simulink model "powertrain_wip_myBatt"  (R2019a)
settings: Solver=VariableStepAuto  StartTime=0.0  StopTime=100  FixedStep=.001  RelTol=1e-3
values from neighbouring files (symbols this model uses):
  Motor =     [current.mat]    (also in rpm.mat; thrust.mat; tout.mat)
undefined symbols (not defined in the file or in its folder): quadModel
libraries: simulink x8
settings Model: Creator=tdarrah  LastModifiedBy=tdarrah
settings DebuggingCC: ArithmeticOperatorsInVariantConditions=warning

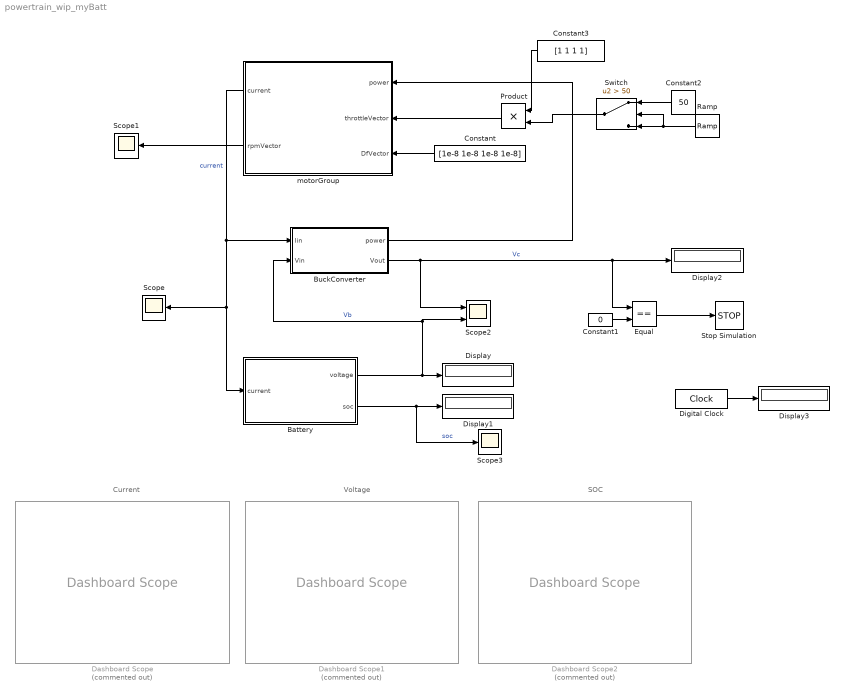
== system powertrain_wip_myBatt ==
  note: Current
  note: Voltage
  note: SOC
  Battery : Subsystem
  BuckConverter : Subsystem
  Constant : Constant  Value=[1e-8 1e-8 1e-8 1e-8]
  Constant1 : Constant  Value=0
  Constant2 : Constant  Value=50
  Constant3 : Constant  Value=[1 1 1 1]
  Dashboard Scope : DashboardScope  Commented=on  Ymin=-5  Ymax=10
  Dashboard Scope1 : DashboardScope  Commented=on  Ymin=8  Ymax=13
  Dashboard Scope2 : DashboardScope  Commented=on
  Digital Clock : DigitalClock
      mask Display: disp('Sim Time');
  Display{,1..3} (4 alike) : Display
  Equal : RelationalOperator  Operator===  OutDataTypeStr=boolean  RndMeth=Simplest
  Product : Product
  Ramp : simulink/Sources/Ramp  slope=1  start=0  InitialOutput=0
  Scope : Scope
  Scope1 : Scope
  Scope2 : Scope  NumInputPorts=2
  Scope3 : Scope
  Stop Simulation : Stop
  Switch : Switch  Criteria=u2 > Threshold  Threshold=50
  motorGroup : Subsystem
  wires:
  Battery/1(voltage) -> BuckConverter/2(Vin), Scope2/2, Display/1  "Vb"
  Battery/2(soc) -> Scope3/1, Display1/1  "soc"
  motorGroup/1(current) -> BuckConverter/1(Iin), Battery/1(current), Scope/1  "current"
  BuckConverter/1(power) -> motorGroup/1(power)
  BuckConverter/2(Vout) -> Scope2/1, Equal/1, Display2/1  "Vc"
  Product/1 -> motorGroup/2(throttleVector)
  Constant/1 -> motorGroup/3(DfVector)
  motorGroup/2(rpmVector) -> Scope1/1
  Constant1/1 -> Equal/2
  Equal/1 -> Stop Simulation/1
  Digital Clock/1 -> Display3/1
  Ramp/1 -> Switch/2, Switch/3
  Constant2/1 -> Switch/1
  Constant3/1 -> Product/1
  Switch/1 -> Product/2

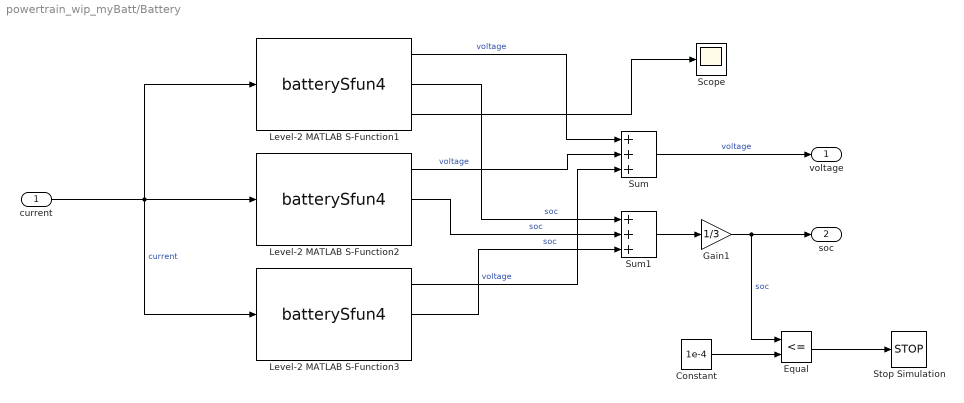
== system powertrain_wip_myBatt/Battery ==
  current : Inport
  Constant : Constant  Value=1e-4
  Equal : RelationalOperator  Operator=<=  OutDataTypeStr=boolean  RndMeth=Simplest
  Gain1 : Gain  Gain=1/3
  Level-2 MATLAB S-Function1 : M-S-Function  FunctionName=batterySfun4  Parameters=battery, soc_ocv, .001
      mask Display:
      | port_label('input', 1, 'current');
      | port_label('output', 1, 'voltage');
      | port_label('output', 2, 'soc');
  Level-2 MATLAB S-Function2 : M-S-Function  FunctionName=batterySfun4  Parameters=battery, soc_ocv, .001
      mask Display:
      | port_label('input', 1, 'current');
      | port_label('output', 1, 'voltage');
      | port_label('output', 2, 'soc');
  Level-2 MATLAB S-Function3 : M-S-Function  FunctionName=batterySfun4  Parameters=battery, soc_ocv, .001
      mask Display:
      | port_label('input', 1, 'current');
      | port_label('output', 1, 'voltage');
      | port_label('output', 2, 'soc');
  Scope : Scope
  Stop Simulation : Stop
  Sum : Sum  Inputs=+++
  Sum1 : Sum  Inputs=+++
  voltage : Outport
  soc : Outport  Port=2
  wires:
  Level-2 MATLAB S-Function2/1 -> Sum/2  "voltage"
  Level-2 MATLAB S-Function1/1 -> Sum/1  "voltage"
  Level-2 MATLAB S-Function2/2 -> Sum1/2  "soc"
  Sum1/1 -> Gain1/1
  Gain1/1 -> Equal/1, soc/1  "soc"
  Level-2 MATLAB S-Function1/2 -> Sum1/1  "soc"
  Level-2 MATLAB S-Function3/2 -> Sum1/3  "soc"
  current/1 -> Level-2 MATLAB S-Function3/1, Level-2 MATLAB S-Function1/1, Level-2 MATLAB S-Function2/1  "current"
  Level-2 MATLAB S-Function3/1 -> Sum/3  "voltage"
  Sum/1 -> voltage/1  "voltage"
  Level-2 MATLAB S-Function1/3 -> Scope/1
  Constant/1 -> Equal/2
  Equal/1 -> Stop Simulation/1

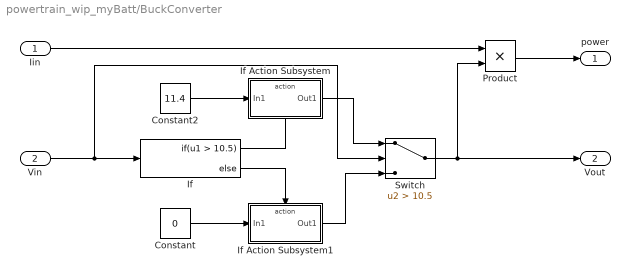
== system powertrain_wip_myBatt/BuckConverter ==
  Iin : Inport
  Vin : Inport  Port=2
  Constant : Constant  Value=0
  Constant2 : Constant  Value=11.4
  If : If  IfExpression=u1 > 10.5
  If Action Subsystem : Subsystem  TreatAsAtomicUnit=on
  If Action Subsystem1 : Subsystem  TreatAsAtomicUnit=on
  Product : Product
  Switch : Switch  Criteria=u2 > Threshold  Threshold=10.5
  power : Outport
  Vout : Outport  Port=2
  wires:
  Product/1 -> power/1
  Iin/1 -> Product/1
  If/1 -> If Action Subsystem/Action
  If/2 -> If Action Subsystem1/Action
  Constant/1 -> If Action Subsystem1/1(In1)
  If Action Subsystem/1(Out1) -> Switch/1
  If Action Subsystem1/1(Out1) -> Switch/3
  Constant2/1 -> If Action Subsystem/1(In1)
  Vin/1 -> Switch/2, If/1
  Switch/1 -> Product/2, Vout/1

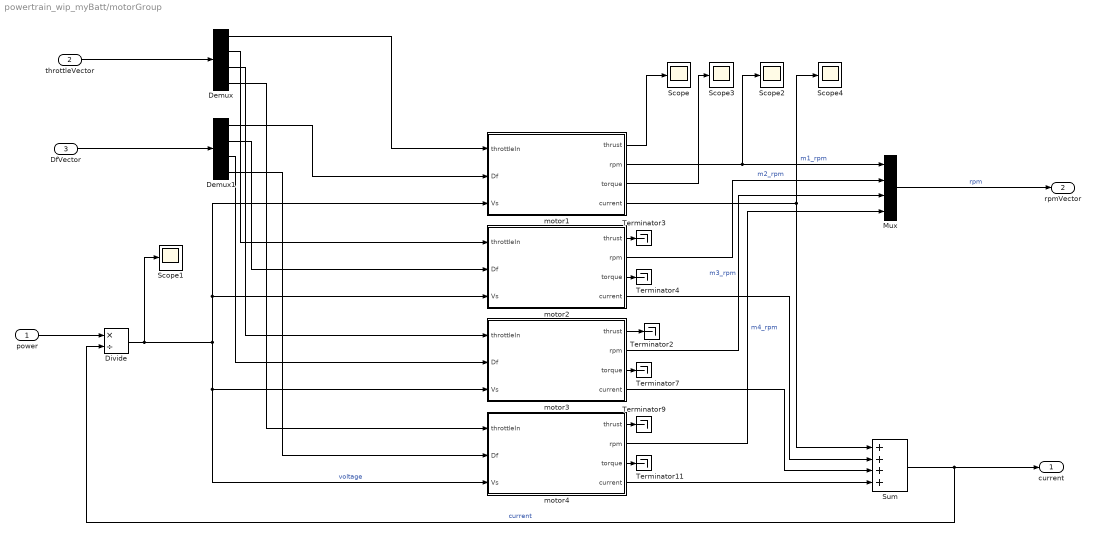
== system powertrain_wip_myBatt/motorGroup ==
  power : Inport
  throttleVector : Inport  Port=2  PortDimensions=4
  DfVector : Inport  Port=3  PortDimensions=4
  Demux : Demux
  Demux1 : Demux
  Divide : Product  Inputs=*/
  Mux : Mux
  Scope{,1..4} (5 alike) : Scope
  Sum : Sum  Inputs=++++
  Terminator{2..4,7,9,11} (6 alike) : Terminator
  motor1 : Subsystem
  motor2 : Subsystem
  motor3 : Subsystem
  motor4 : Subsystem
  current : Outport
  rpmVector : Outport  Port=2
  wires:
  Demux1/2 -> motor2/2(Df)
  Demux1/4 -> motor4/2(Df)
  Divide/1 -> Scope1/1, motor1/3(Vs), motor2/3(Vs), motor4/3(Vs), motor3/3(Vs)  "voltage"
  Demux1/1 -> motor1/2(Df)
  Sum/1 -> current/1, Divide/2  "current"
  Demux1/3 -> motor3/2(Df)
  motor1/4(current) -> Scope4/1, Sum/1
  power/1 -> Divide/1
  Demux/4 -> motor4/1(throttleIn)
  Demux/3 -> motor3/1(throttleIn)
  Demux/2 -> motor2/1(throttleIn)
  Demux/1 -> motor1/1(throttleIn)
  throttleVector/1 -> Demux/1
  DfVector/1 -> Demux1/1
  motor4/4(current) -> Sum/4
  motor3/4(current) -> Sum/3
  motor2/4(current) -> Sum/2
  motor4/2(rpm) -> Mux/4  "m4_rpm"
  motor3/2(rpm) -> Mux/3  "m3_rpm"
  motor2/2(rpm) -> Mux/2  "m2_rpm"
  motor1/2(rpm) -> Scope2/1, Mux/1  "m1_rpm"
  Mux/1 -> rpmVector/1  "rpm"
  motor1/1(thrust) -> Scope/1
  motor4/3(torque) -> Terminator11/1
  motor1/3(torque) -> Scope3/1
  motor2/3(torque) -> Terminator4/1
  motor3/3(torque) -> Terminator7/1
  motor4/1(thrust) -> Terminator9/1
  motor3/1(thrust) -> Terminator2/1
  motor2/1(thrust) -> Terminator3/1

== system powertrain_wip_myBatt/BuckConverter/If Action Subsystem ==
  In1 : Inport
  Action Port : ActionPort  ActionPortLabel=if(u1 > 10.5)
  Out1 : Outport
  wires:
  In1/1 -> Out1/1

== system powertrain_wip_myBatt/BuckConverter/If Action Subsystem1 ==
  In1 : Inport
  Action Port : ActionPort  ActionPortLabel=else
  Out1 : Outport
  wires:
  In1/1 -> Out1/1

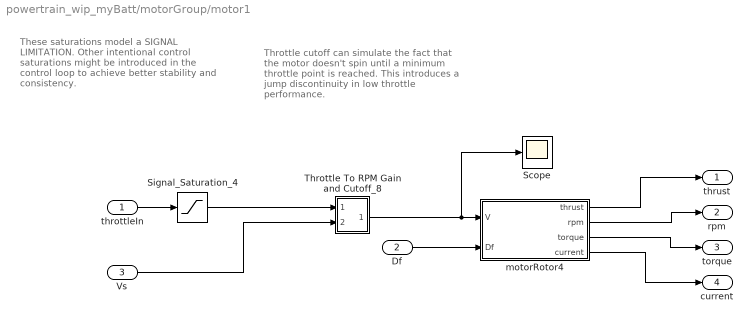
== system powertrain_wip_myBatt/motorGroup/motor1 ==
  note: Throttle cutoff can simulate the fact that the motor doesn't
      | spin until a minimum throttle point is reached. This introduces
      | a jump discontinuity in low throttle performance.
  note: These saturations model a SIGNAL LIMITATION.
      | Other intentional control saturations might be introduced in the
      | control loop to achieve better stability and consistency.
  throttleIn : Inport
  Df : Inport  Port=2
  Vs : Inport  Port=3
  Scope : Scope
  Signal_Saturation_4 : Saturate  UpperLimit=100  LowerLimit=0
  Throttle To RPM Gain and Cutoff_8 : Subsystem
  motorRotor4 : Subsystem
  thrust : Outport
  rpm : Outport  Port=2
  torque : Outport  Port=3
  current : Outport  Port=4
  wires:
  Throttle To RPM Gain and Cutoff_8/1(Out5) -> motorRotor4/1(V), Scope/1
  motorRotor4/4(current) -> current/1
  motorRotor4/2(rpm) -> rpm/1
  throttleIn/1 -> Signal_Saturation_4/1
  motorRotor4/3(torque) -> torque/1
  motorRotor4/1(thrust) -> thrust/1
  Signal_Saturation_4/1 -> Throttle To RPM Gain and Cutoff_8/1(In5)
  Df/1 -> motorRotor4/2(Df)
  Vs/1 -> Throttle To RPM Gain and Cutoff_8/2(Vs)

== system powertrain_wip_myBatt/motorGroup/motor2 ==
  note: Throttle cutoff can simulate the fact that the motor doesn't
      | spin until a minimum throttle point is reached. This introduces
      | a jump discontinuity in low throttle performance.
  note: These saturations model a SIGNAL LIMITATION.
      | Other intentional control saturations might be introduced in the
      | control loop to achieve better stability and consistency.
  throttleIn : Inport
  Df : Inport  Port=2
  Vs : Inport  Port=3
  Scope : Scope
  Signal_Saturation_4 : Saturate  UpperLimit=100  LowerLimit=0
  Throttle To RPM Gain and Cutoff_8 : Subsystem
  motorRotor4 : Subsystem
  thrust : Outport
  rpm : Outport  Port=2
  torque : Outport  Port=3
  current : Outport  Port=4
  wires:
  Throttle To RPM Gain and Cutoff_8/1(Out5) -> motorRotor4/1(V), Scope/1
  motorRotor4/4(current) -> current/1
  motorRotor4/2(rpm) -> rpm/1
  throttleIn/1 -> Signal_Saturation_4/1
  motorRotor4/3(torque) -> torque/1
  motorRotor4/1(thrust) -> thrust/1
  Signal_Saturation_4/1 -> Throttle To RPM Gain and Cutoff_8/1(In5)
  Df/1 -> motorRotor4/2(Df)
  Vs/1 -> Throttle To RPM Gain and Cutoff_8/2(Vs)

== system powertrain_wip_myBatt/motorGroup/motor3 ==
  note: Throttle cutoff can simulate the fact that the motor doesn't
      | spin until a minimum throttle point is reached. This introduces
      | a jump discontinuity in low throttle performance.
  note: These saturations model a SIGNAL LIMITATION.
      | Other intentional control saturations might be introduced in the
      | control loop to achieve better stability and consistency.
  throttleIn : Inport
  Df : Inport  Port=2
  Vs : Inport  Port=3
  Scope : Scope
  Signal_Saturation_4 : Saturate  UpperLimit=100  LowerLimit=0
  Throttle To RPM Gain and Cutoff_8 : Subsystem
  motorRotor4 : Subsystem
  thrust : Outport
  rpm : Outport  Port=2
  torque : Outport  Port=3
  current : Outport  Port=4
  wires:
  Throttle To RPM Gain and Cutoff_8/1(Out5) -> motorRotor4/1(V), Scope/1
  motorRotor4/4(current) -> current/1
  motorRotor4/2(rpm) -> rpm/1
  throttleIn/1 -> Signal_Saturation_4/1
  motorRotor4/3(torque) -> torque/1
  motorRotor4/1(thrust) -> thrust/1
  Signal_Saturation_4/1 -> Throttle To RPM Gain and Cutoff_8/1(In5)
  Df/1 -> motorRotor4/2(Df)
  Vs/1 -> Throttle To RPM Gain and Cutoff_8/2(Vs)

== system powertrain_wip_myBatt/motorGroup/motor4 ==
  note: Throttle cutoff can simulate the fact that the motor doesn't
      | spin until a minimum throttle point is reached. This introduces
      | a jump discontinuity in low throttle performance.
  note: These saturations model a SIGNAL LIMITATION.
      | Other intentional control saturations might be introduced in the
      | control loop to achieve better stability and consistency.
  throttleIn : Inport
  Df : Inport  Port=2
  Vs : Inport  Port=3
  Scope : Scope
  Signal_Saturation_4 : Saturate  UpperLimit=100  LowerLimit=0
  Throttle To RPM Gain and Cutoff_8 : Subsystem
  motorRotor4 : Subsystem
  thrust : Outport
  rpm : Outport  Port=2
  torque : Outport  Port=3
  current : Outport  Port=4
  wires:
  Throttle To RPM Gain and Cutoff_8/1(Out5) -> motorRotor4/1(V), Scope/1
  motorRotor4/4(current) -> current/1
  motorRotor4/2(rpm) -> rpm/1
  throttleIn/1 -> Signal_Saturation_4/1
  motorRotor4/3(torque) -> torque/1
  motorRotor4/1(thrust) -> thrust/1
  Signal_Saturation_4/1 -> Throttle To RPM Gain and Cutoff_8/1(In5)
  Df/1 -> motorRotor4/2(Df)
  Vs/1 -> Throttle To RPM Gain and Cutoff_8/2(Vs)

== system powertrain_wip_myBatt/motorGroup/motor1/Throttle To RPM Gain and Cutoff_8 ==
  note: Output equals linearly scaled RPM
      | for given throttle input if throttle input >=Throttle Cuttoff (minThr)
      | else output is zero.
  In5 : Inport
  Vs : Inport  Port=2
  Gain : Gain  Gain=.01
  Minimum Throttle Cutoff : simulink/Logic and Bit Operations/Compare To Constant  relop=>=  const=5  OutDataTypeStr=uint8
  Product : Product
  Product2 : Product
  Out5 : Outport
  wires:
  Minimum Throttle Cutoff/1 -> Product/2
  Product/1 -> Out5/1
  In5/1 -> Gain/1, Minimum Throttle Cutoff/1
  Gain/1 -> Product2/2
  Product2/1 -> Product/1
  Vs/1 -> Product2/1

== system powertrain_wip_myBatt/motorGroup/motor1/motorRotor4 ==
  V : Inport
  Df : Inport  Port=2
  Electrical part : Subsystem
  Mechanical part : Subsystem
  thrust : Outport
  rpm : Outport  Port=2
  torque : Outport  Port=3
  current : Outport  Port=4
  wires:
  V/1 -> Electrical part/1(Vin)
  Mechanical part/2(Thrust) -> thrust/1
  Electrical part/1(Electrical Torque) -> Mechanical part/2(Electrical Torque)
  Mechanical part/4(Torque) -> torque/1
  Mechanical part/1(w angular speed) -> Electrical part/2(w angular speed)
  Df/1 -> Mechanical part/1(dynamicFriction)
  Electrical part/2(current) -> current/1
  Mechanical part/3(rpm) -> rpm/1

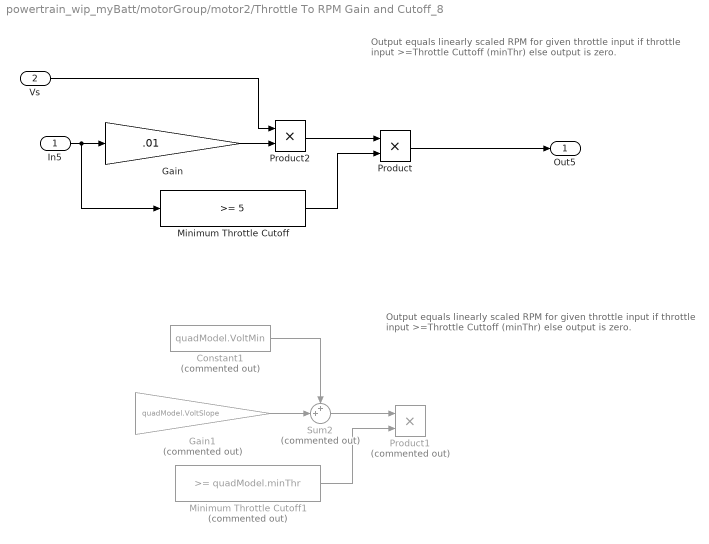
== system powertrain_wip_myBatt/motorGroup/motor2/Throttle To RPM Gain and Cutoff_8 ==
  note: Output equals linearly scaled RPM
      | for given throttle input if throttle input >=Throttle Cuttoff (minThr)
      | else output is zero.
  note: Output equals linearly scaled RPM
      | for given throttle input if throttle input >=Throttle Cuttoff (minThr)
      | else output is zero.
  In5 : Inport
  Vs : Inport  Port=2
  Constant1 : Constant  Commented=on  Value=quadModel.VoltMin
  Gain : Gain  Gain=.01
  Gain1 : Gain  Commented=on  Gain=quadModel.VoltSlope
  Minimum Throttle Cutoff : simulink/Logic and Bit Operations/Compare To Constant  relop=>=  const=5  OutDataTypeStr=uint8
  Minimum Throttle Cutoff1 : simulink/Logic and Bit Operations/Compare To Constant  Commented=on  relop=>=  const=quadModel.minThr  OutDataTypeStr=uint8
  Product : Product
  Product1 : Product  Commented=on
  Product2 : Product
  Sum2 : Sum  Commented=on  Inputs=++|
  Out5 : Outport
  wires:
  Minimum Throttle Cutoff/1 -> Product/2
  Product/1 -> Out5/1
  In5/1 -> Gain/1, Minimum Throttle Cutoff/1
  Gain/1 -> Product2/2
  Product2/1 -> Product/1
  Gain1/1 -> Sum2/2
  Constant1/1 -> Sum2/1
  Sum2/1 -> Product1/1
  Minimum Throttle Cutoff1/1 -> Product1/2
  Vs/1 -> Product2/1

== system powertrain_wip_myBatt/motorGroup/motor2/motorRotor4 ==
  V : Inport
  Df : Inport  Port=2
  Convert rad/s to rmp : Gain  Gain=60/(2*pi)
  Electrical part : Subsystem
  Mechanical part : Subsystem
  thrust : Outport
  rpm : Outport  Port=2
  torque : Outport  Port=3
  current : Outport  Port=4
  wires:
  Convert rad/s to rmp/1 -> rpm/1
  V/1 -> Electrical part/1(ESC voltage)
  Mechanical part/2(Thrust) -> thrust/1
  Electrical part/1(Electrical Torque) -> Mechanical part/2(Electrical Torque)
  Mechanical part/3(Torque) -> torque/1
  Mechanical part/1(w angular speed) -> Electrical part/2(w angular speed), Convert rad/s to rmp/1
  Df/1 -> Mechanical part/1(dynamicFriction)
  Electrical part/2(current) -> current/1

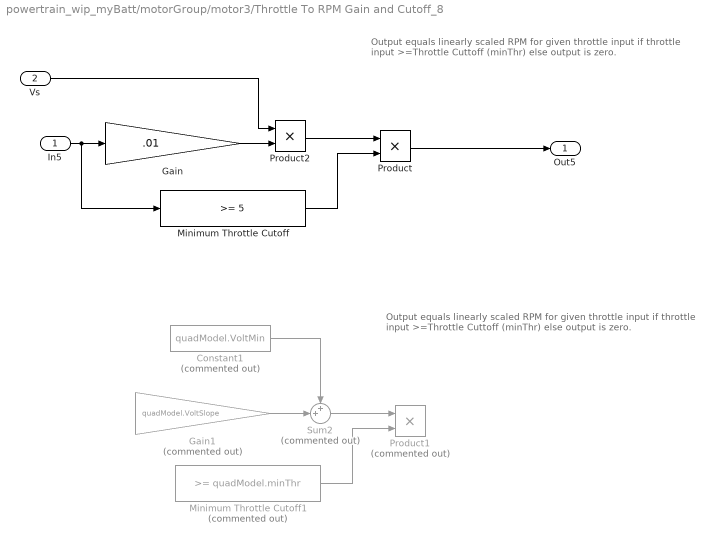
== system powertrain_wip_myBatt/motorGroup/motor3/Throttle To RPM Gain and Cutoff_8 ==
  note: Output equals linearly scaled RPM
      | for given throttle input if throttle input >=Throttle Cuttoff (minThr)
      | else output is zero.
  note: Output equals linearly scaled RPM
      | for given throttle input if throttle input >=Throttle Cuttoff (minThr)
      | else output is zero.
  In5 : Inport
  Vs : Inport  Port=2
  Constant1 : Constant  Commented=on  Value=quadModel.VoltMin
  Gain : Gain  Gain=.01
  Gain1 : Gain  Commented=on  Gain=quadModel.VoltSlope
  Minimum Throttle Cutoff : simulink/Logic and Bit Operations/Compare To Constant  relop=>=  const=5  OutDataTypeStr=uint8
  Minimum Throttle Cutoff1 : simulink/Logic and Bit Operations/Compare To Constant  Commented=on  relop=>=  const=quadModel.minThr  OutDataTypeStr=uint8
  Product : Product
  Product1 : Product  Commented=on
  Product2 : Product
  Sum2 : Sum  Commented=on  Inputs=++|
  Out5 : Outport
  wires:
  Minimum Throttle Cutoff/1 -> Product/2
  Product/1 -> Out5/1
  In5/1 -> Gain/1, Minimum Throttle Cutoff/1
  Gain/1 -> Product2/2
  Product2/1 -> Product/1
  Gain1/1 -> Sum2/2
  Constant1/1 -> Sum2/1
  Sum2/1 -> Product1/1
  Minimum Throttle Cutoff1/1 -> Product1/2
  Vs/1 -> Product2/1

== system powertrain_wip_myBatt/motorGroup/motor3/motorRotor4 ==
  V : Inport
  Df : Inport  Port=2
  Convert rad/s to rmp : Gain  Gain=60/(2*pi)
  Electrical part : Subsystem
  Mechanical part : Subsystem
  thrust : Outport
  rpm : Outport  Port=2
  torque : Outport  Port=3
  current : Outport  Port=4
  wires:
  Convert rad/s to rmp/1 -> rpm/1
  V/1 -> Electrical part/1(ESC voltage)
  Mechanical part/2(Thrust) -> thrust/1
  Electrical part/1(Electrical Torque) -> Mechanical part/2(Electrical Torque)
  Mechanical part/3(Torque) -> torque/1
  Mechanical part/1(w angular speed) -> Electrical part/2(w angular speed), Convert rad/s to rmp/1
  Df/1 -> Mechanical part/1(dynamicFriction)
  Electrical part/2(current) -> current/1

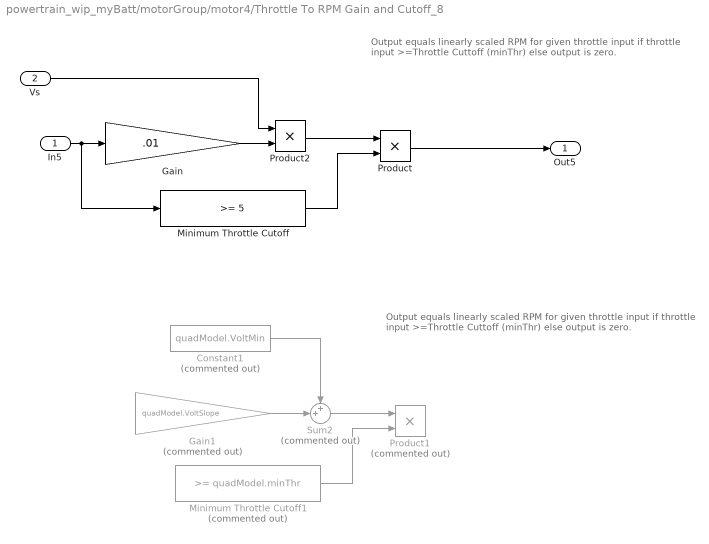
== system powertrain_wip_myBatt/motorGroup/motor4/Throttle To RPM Gain and Cutoff_8 ==
  note: Output equals linearly scaled RPM
      | for given throttle input if throttle input >=Throttle Cuttoff (minThr)
      | else output is zero.
  note: Output equals linearly scaled RPM
      | for given throttle input if throttle input >=Throttle Cuttoff (minThr)
      | else output is zero.
  In5 : Inport
  Vs : Inport  Port=2
  Constant1 : Constant  Commented=on  Value=quadModel.VoltMin
  Gain : Gain  Gain=.01
  Gain1 : Gain  Commented=on  Gain=quadModel.VoltSlope
  Minimum Throttle Cutoff : simulink/Logic and Bit Operations/Compare To Constant  relop=>=  const=5  OutDataTypeStr=uint8
  Minimum Throttle Cutoff1 : simulink/Logic and Bit Operations/Compare To Constant  Commented=on  relop=>=  const=quadModel.minThr  OutDataTypeStr=uint8
  Product : Product
  Product1 : Product  Commented=on
  Product2 : Product
  Sum2 : Sum  Commented=on  Inputs=++|
  Out5 : Outport
  wires:
  Minimum Throttle Cutoff/1 -> Product/2
  Product/1 -> Out5/1
  In5/1 -> Gain/1, Minimum Throttle Cutoff/1
  Gain/1 -> Product2/2
  Product2/1 -> Product/1
  Gain1/1 -> Sum2/2
  Constant1/1 -> Sum2/1
  Sum2/1 -> Product1/1
  Minimum Throttle Cutoff1/1 -> Product1/2
  Vs/1 -> Product2/1

== system powertrain_wip_myBatt/motorGroup/motor4/motorRotor4 ==
  V : Inport
  Df : Inport  Port=2
  Convert rad/s to rmp : Gain  Gain=60/(2*pi)
  Electrical part : Subsystem
  Mechanical part : Subsystem
  thrust : Outport
  rpm : Outport  Port=2
  torque : Outport  Port=3
  current : Outport  Port=4
  wires:
  Convert rad/s to rmp/1 -> rpm/1
  V/1 -> Electrical part/1(ESC voltage)
  Mechanical part/2(Thrust) -> thrust/1
  Electrical part/1(Electrical Torque) -> Mechanical part/2(Electrical Torque)
  Mechanical part/3(Torque) -> torque/1
  Mechanical part/1(w angular speed) -> Electrical part/2(w angular speed), Convert rad/s to rmp/1
  Df/1 -> Mechanical part/1(dynamicFriction)
  Electrical part/2(current) -> current/1

== system powertrain_wip_myBatt/motorGroup/motor1/motorRotor4/Electrical part ==
  Vin : Inport
  w angular speed : Inport  Port=2
  1/R : Gain  Gain=1/Motor.Req
  Ke (Torque constant)1 : Gain  Gain=Motor.Ke_eq
  Kt (Torque constant) Kt=Ke for an ideal square wave motor : Gain  Gain=Motor.Ke_eq
  Sum : Sum  Inputs=|+-
  Electrical Torque : Outport
  current : Outport  Port=2
  wires:
  1/R/1 -> current/1, Kt (Torque constant) Kt=Ke for an ideal square wave motor/1  "current i"
  Sum/1 -> 1/R/1
  Kt (Torque constant) Kt=Ke for an ideal square wave motor/1 -> Electrical Torque/1
  Ke (Torque constant)1/1 -> Sum/2
  Vin/1 -> Sum/1
  w angular speed/1 -> Ke (Torque constant)1/1

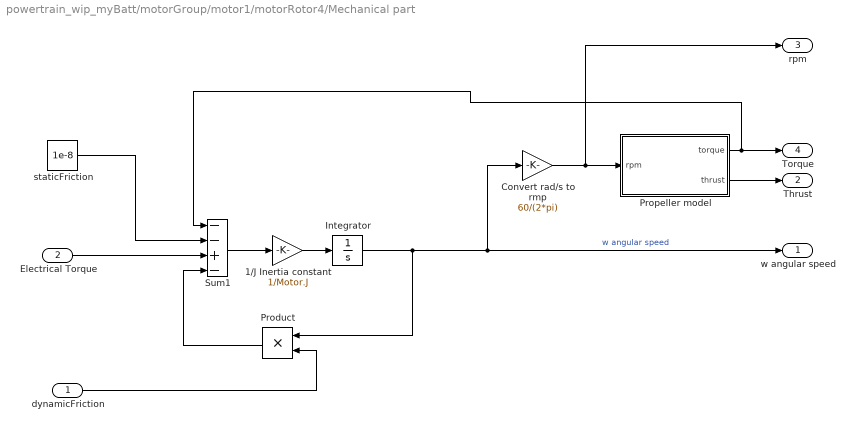
== system powertrain_wip_myBatt/motorGroup/motor1/motorRotor4/Mechanical part ==
  dynamicFriction : Inport
  Electrical Torque : Inport  Port=2
  1/J Inertia constant : Gain  Gain=1/Motor.J
  Convert rad/s to rmp : Gain  Gain=60/(2*pi)
  Integrator : Integrator  InitialCondition=419
  Product : Product
  "Propeller model " : MATLAB Function  TreatAsAtomicUnit=on
  Sum1 : Sum  Inputs=--+-
  staticFriction : Constant  Value=1e-8
  w angular speed : Outport
  Thrust : Outport  Port=2
  rpm : Outport  Port=3
  Torque : Outport  Port=4
  wires:
  "Propeller model "/1(torque) -> Sum1/1, Torque/1
  1/J Inertia constant/1 -> Integrator/1
  dynamicFriction/1 -> Product/2
  Product/1 -> Sum1/4
  Integrator/1 -> Product/1, w angular speed/1, Convert rad/s to rmp/1  "w angular speed"
  Sum1/1 -> 1/J Inertia constant/1
  Electrical Torque/1 -> Sum1/3
  Convert rad/s to rmp/1 -> rpm/1, "Propeller model "/1(rpm)
  "Propeller model "/2(thrust) -> Thrust/1
  staticFriction/1 -> Sum1/2

== system powertrain_wip_myBatt/motorGroup/motor2/motorRotor4/Electrical part ==
  ESC voltage : Inport
  w angular speed : Inport  Port=2
  1/R : Gain  Gain=1/Motor.Req
  Ke (Torque constant)1 : Gain  Gain=Motor.Ke_eq
  Kt (Torque constant) Kt=Ke for an ideal square wave motor : Gain  Gain=Motor.Ke_eq
  Sum : Sum  Inputs=|+-
  Electrical Torque : Outport
  current : Outport  Port=2
  wires:
  1/R/1 -> current/1, Kt (Torque constant) Kt=Ke for an ideal square wave motor/1  "current i"
  Sum/1 -> 1/R/1
  Kt (Torque constant) Kt=Ke for an ideal square wave motor/1 -> Electrical Torque/1
  Ke (Torque constant)1/1 -> Sum/2
  ESC voltage/1 -> Sum/1
  w angular speed/1 -> Ke (Torque constant)1/1

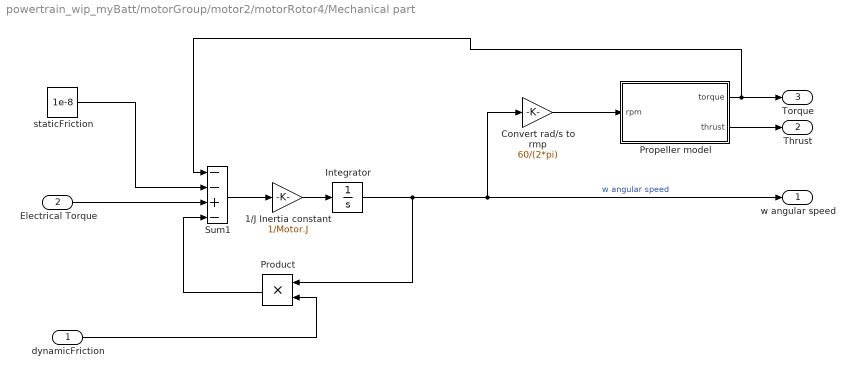
== system powertrain_wip_myBatt/motorGroup/motor2/motorRotor4/Mechanical part ==
  dynamicFriction : Inport
  Electrical Torque : Inport  Port=2
  1/J Inertia constant : Gain  Gain=1/Motor.J
  Convert rad/s to rmp : Gain  Gain=60/(2*pi)
  Integrator : Integrator  InitialCondition=419
  Product : Product
  "Propeller model " : MATLAB Function  TreatAsAtomicUnit=on
  Sum1 : Sum  Inputs=--+-
  staticFriction : Constant  Value=1e-8
  w angular speed : Outport
  Thrust : Outport  Port=2
  Torque : Outport  Port=3
  wires:
  "Propeller model "/1(torque) -> Sum1/1, Torque/1
  1/J Inertia constant/1 -> Integrator/1
  dynamicFriction/1 -> Product/2
  Product/1 -> Sum1/4
  Integrator/1 -> Product/1, w angular speed/1, Convert rad/s to rmp/1  "w angular speed"
  Sum1/1 -> 1/J Inertia constant/1
  Electrical Torque/1 -> Sum1/3
  Convert rad/s to rmp/1 -> "Propeller model "/1(rpm)
  "Propeller model "/2(thrust) -> Thrust/1
  staticFriction/1 -> Sum1/2

== system powertrain_wip_myBatt/motorGroup/motor3/motorRotor4/Electrical part ==
  ESC voltage : Inport
  w angular speed : Inport  Port=2
  1/R : Gain  Gain=1/Motor.Req
  Ke (Torque constant)1 : Gain  Gain=Motor.Ke_eq
  Kt (Torque constant) Kt=Ke for an ideal square wave motor : Gain  Gain=Motor.Ke_eq
  Sum : Sum  Inputs=|+-
  Electrical Torque : Outport
  current : Outport  Port=2
  wires:
  1/R/1 -> current/1, Kt (Torque constant) Kt=Ke for an ideal square wave motor/1  "current i"
  Sum/1 -> 1/R/1
  Kt (Torque constant) Kt=Ke for an ideal square wave motor/1 -> Electrical Torque/1
  Ke (Torque constant)1/1 -> Sum/2
  ESC voltage/1 -> Sum/1
  w angular speed/1 -> Ke (Torque constant)1/1

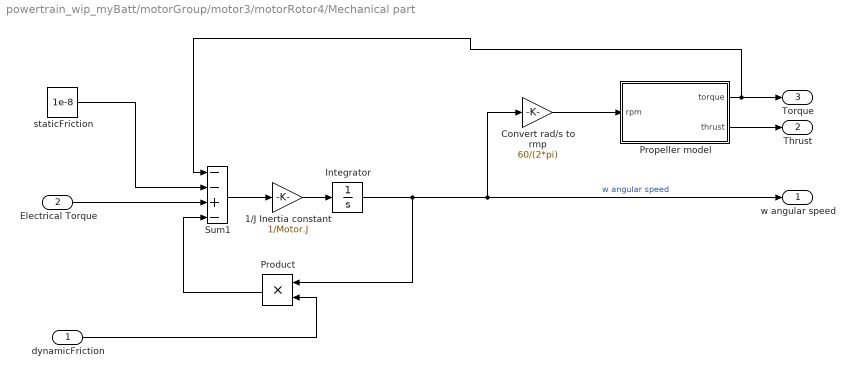
== system powertrain_wip_myBatt/motorGroup/motor3/motorRotor4/Mechanical part ==
  dynamicFriction : Inport
  Electrical Torque : Inport  Port=2
  1/J Inertia constant : Gain  Gain=1/Motor.J
  Convert rad/s to rmp : Gain  Gain=60/(2*pi)
  Integrator : Integrator  InitialCondition=419
  Product : Product
  "Propeller model " : MATLAB Function  TreatAsAtomicUnit=on
  Sum1 : Sum  Inputs=--+-
  staticFriction : Constant  Value=1e-8
  w angular speed : Outport
  Thrust : Outport  Port=2
  Torque : Outport  Port=3
  wires:
  "Propeller model "/1(torque) -> Sum1/1, Torque/1
  1/J Inertia constant/1 -> Integrator/1
  dynamicFriction/1 -> Product/2
  Product/1 -> Sum1/4
  Integrator/1 -> Product/1, w angular speed/1, Convert rad/s to rmp/1  "w angular speed"
  Sum1/1 -> 1/J Inertia constant/1
  Electrical Torque/1 -> Sum1/3
  Convert rad/s to rmp/1 -> "Propeller model "/1(rpm)
  "Propeller model "/2(thrust) -> Thrust/1
  staticFriction/1 -> Sum1/2

== system powertrain_wip_myBatt/motorGroup/motor4/motorRotor4/Electrical part ==
  ESC voltage : Inport
  w angular speed : Inport  Port=2
  1/R : Gain  Gain=1/Motor.Req
  Ke (Torque constant)1 : Gain  Gain=Motor.Ke_eq
  Kt (Torque constant) Kt=Ke for an ideal square wave motor : Gain  Gain=Motor.Ke_eq
  Sum : Sum  Inputs=|+-
  Electrical Torque : Outport
  current : Outport  Port=2
  wires:
  1/R/1 -> current/1, Kt (Torque constant) Kt=Ke for an ideal square wave motor/1  "current i"
  Sum/1 -> 1/R/1
  Kt (Torque constant) Kt=Ke for an ideal square wave motor/1 -> Electrical Torque/1
  Ke (Torque constant)1/1 -> Sum/2
  ESC voltage/1 -> Sum/1
  w angular speed/1 -> Ke (Torque constant)1/1

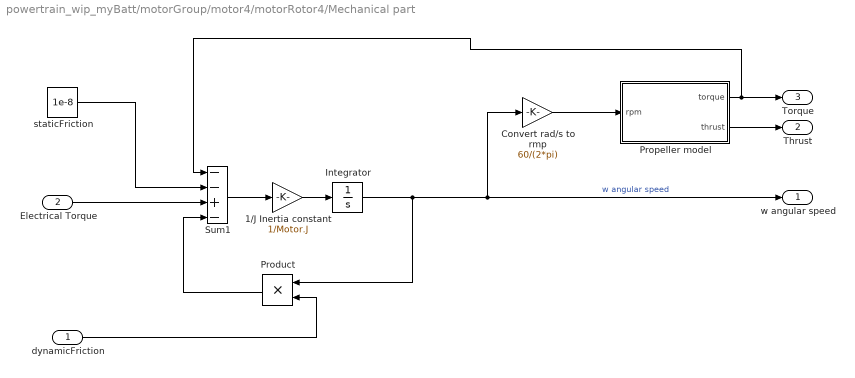
== system powertrain_wip_myBatt/motorGroup/motor4/motorRotor4/Mechanical part ==
  dynamicFriction : Inport
  Electrical Torque : Inport  Port=2
  1/J Inertia constant : Gain  Gain=1/Motor.J
  Convert rad/s to rmp : Gain  Gain=60/(2*pi)
  Integrator : Integrator  InitialCondition=419
  Product : Product
  "Propeller model " : MATLAB Function  TreatAsAtomicUnit=on
  Sum1 : Sum  Inputs=--+-
  staticFriction : Constant  Value=1e-8
  w angular speed : Outport
  Thrust : Outport  Port=2
  Torque : Outport  Port=3
  wires:
  "Propeller model "/1(torque) -> Sum1/1, Torque/1
  1/J Inertia constant/1 -> Integrator/1
  dynamicFriction/1 -> Product/2
  Product/1 -> Sum1/4
  Integrator/1 -> Product/1, w angular speed/1, Convert rad/s to rmp/1  "w angular speed"
  Sum1/1 -> 1/J Inertia constant/1
  Electrical Torque/1 -> Sum1/3
  Convert rad/s to rmp/1 -> "Propeller model "/1(rpm)
  "Propeller model "/2(thrust) -> Thrust/1
  staticFriction/1 -> Sum1/2

== matlab function powertrain_wip_myBatt/motorGroup/motor1/motorRotor4/Mechanical part/Propeller model  ==
  data: torque output; rpm input; thrust output
function [torque,thrust] = fcn(rpm)
% angular_velocity in rpm

%coefficient of thrust, empirically derived
coef_t = 2*(10^-15)*rpm^3 - 4*(10^-11)*rpm^2 + 3*(10^-7)*rpm + .1013;
%thrust = coef_t * density of air * velocity^2 * propeller diameter (m) ^4
thrust = coef_t*1.225*(rpm/60)^2*.2^4;
% empirically derived
torque = 4*(10^-14)*rpm^3 +  8*(10^-12)*rpm^2 + 3*(10^-6)*rpm;
end

== matlab function powertrain_wip_myBatt/motorGroup/motor2/motorRotor4/Mechanical part/Propeller model  ==
  data: torque output; rpm input; thrust output
function [torque,thrust] = fcn(rpm)
% angular_velocity in rpm

%coefficient of thrust, empirically derived
coef_t = 2*(10^-15)*rpm^3 - 4*(10^-11)*rpm^2 + 3*(10^-7)*rpm + .1013;
%thrust = coef_t * density of air * velocity^2 * propeller diameter (m) ^4
thrust = coef_t*1.225*(rpm/60)^2*.2^4;
% empirically derived
torque = 4*(10^-14)*rpm^3 +  8*(10^-12)*rpm^2 + 3*(10^-6)*rpm;
end

== matlab function powertrain_wip_myBatt/motorGroup/motor3/motorRotor4/Mechanical part/Propeller model  ==
  data: torque output; rpm input; thrust output
function [torque,thrust] = fcn(rpm)
% angular_velocity in rpm

%coefficient of thrust, empirically derived
coef_t = 2*(10^-15)*rpm^3 - 4*(10^-11)*rpm^2 + 3*(10^-7)*rpm + .1013;
%thrust = coef_t * density of air * velocity^2 * propeller diameter (m) ^4
thrust = coef_t*1.225*(rpm/60)^2*.2^4;
% empirically derived
torque = 4*(10^-14)*rpm^3 +  8*(10^-12)*rpm^2 + 3*(10^-6)*rpm;
end

== matlab function powertrain_wip_myBatt/motorGroup/motor4/motorRotor4/Mechanical part/Propeller model  ==
  data: torque output; rpm input; thrust output
function [torque,thrust] = fcn(rpm)
% angular_velocity in rpm

%coefficient of thrust, empirically derived
coef_t = 2*(10^-15)*rpm^3 - 4*(10^-11)*rpm^2 + 3*(10^-7)*rpm + .1013;
%thrust = coef_t * density of air * velocity^2 * propeller diameter (m) ^4
thrust = coef_t*1.225*(rpm/60)^2*.2^4;
% empirically derived
torque = 4*(10^-14)*rpm^3 +  8*(10^-12)*rpm^2 + 3*(10^-6)*rpm;
end
